simulink model "obstacle_detection"  (R2023a)
settings: Solver=ode1  StartTime=0.0  StopTime=Inf  FixedStep=1/60  RelTol=1e-3
PostLoadFcn:
  | qlabs_setup
model workspace (MAT data in the model file):
  downCamStepSize = Simulink.Parameter
  downCamStepSize.Value = Simulink.data.Expression
  downCamStepSize.Value.ExpressionString = "qc_get_step_size*ceil(1/60/qc_get_step_size)"
  downCamStepSize.DataType = 'auto'
  downCamStepSize.Complexity = 'real'
  downCamStepSize.Dimensions = -1
  lidarStepSize = Simulink.Parameter
  lidarStepSize.Value = Simulink.data.Expression
  lidarStepSize.Value.ExpressionString = "qc_get_step_size*ceil(1/5/qc_get_step_size)"
  lidarStepSize.DataType = 'auto'
  lidarStepSize.Complexity = 'real'
  lidarStepSize.Dimensions = -1
  mainStepSize = Simulink.Parameter
  mainStepSize.Value = Simulink.data.Expression
  mainStepSize.Value.ExpressionString = "qc_get_step_size"
  mainStepSize.DataType = 'auto'
  mainStepSize.Complexity = 'real'
  mainStepSize.Dimensions = -1
  mode = Simulink.Parameter
  mode.Value = 1
  mode.Description = '0 - education speeds via wheel speed commands
    | 1 - education speeds via body speed commands
    | 2 - research speeds via wheel speed commands
    | 3 - research speeds via body speed commands'
  mode.DataType = 'auto'
  mode.Complexity = 'real'
  mode.Dimensions = [1 1]
  realSenseStepSize = Simulink.Parameter
  realSenseStepSize.Value = Simulink.data.Expression
  realSenseStepSize.Value.ExpressionString = "qc_get_step_size*ceil(1/30/qc_get_step_size)"
  realSenseStepSize.DataType = 'auto'
  realSenseStepSize.Complexity = 'real'
  realSenseStepSize.Dimensions = -1
undefined symbols (not defined in the file or in its folder): gcbh, JPEG, Point, video_display_show
libraries: quarc_library x29
settings Model: SimulationMode=external  ExtModeTrigDuration=10000  Creator=mbohra  LastModifiedBy=ZinanCen
settings DebuggingCC: UnderspecifiedInitializationDetection=Classic  MergeDetectMultiDrivingBlocksExec=none
settings ModelReferenceCC: PropagateSignalLabelsOutOfModel=off

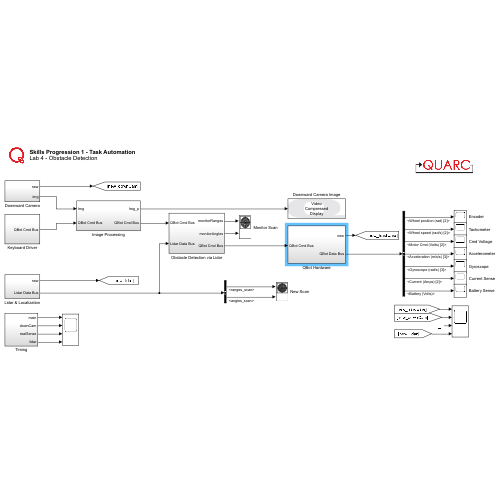
[thumbnail: Simulink's stored preview of the top-level diagram]
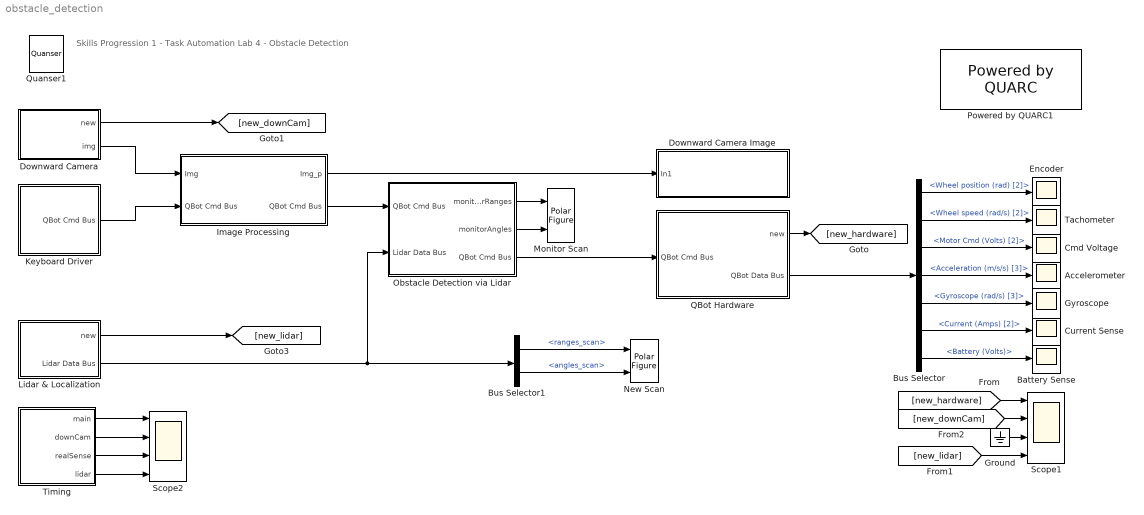
== system obstacle_detection ==
  note: Skills Progression 1 - Task Automation
      | Lab 4 - Obstacle Detection
  Accelerometer : Scope
  Battery Sense : Scope
  Bus Selector : BusSelector  OutputSignals=Wheel position (rad) [2],Wheel speed (rad/s) [2],Motor Cmd (Volts) [2],Acceleration (m/s/s) [3],Gyroscope (rad/s) [3],Current (Amps) [2],Battery (Volts)
  Bus Selector1 : BusSelector  OutputSignals=ranges_scan,angles_scan
  Cmd Voltage : Scope
  Current Sense : Scope
  Downward Camera : Subsystem
  Downward Camera Image : Subsystem  LoadFcn=set_param(gcbh, 'UserData', gcb);  StartFcn=video_display_show([gcb, '/Video Display'], 'add', gcb);  mask(Video Compressed Display){algorithm=JPEG, quality=50, sample_time=-1, use_hardware=on}
      mask prompts: algorithm "Compression algorithm:"; quality "Compression quality (0-100):"; sample_time "Sample time (seconds):"; use_hardware "Use hardware acceleration for video display"
      mask help: Displays a video stream on the host, using compression to minimize bandwidth.
      mask init:
      | qc_set_display('Video\nCompressed\nDisplay');
      settings: UndoDeleteFcn=set_param(gcbh, 'UserData', gcb);  OpenFcn=video_display_show([gcb, '/Video Display'], 'show', gcb);  PreDeleteFcn=video_display_show([gcb, '/Video Display'], 'delete');
      settings: CopyFcn=|
      | set_param(gcbh, 'UserData', gcb);
      | set_param(gcbh, 'LinkStatus', 'none');
      settings: NameChangeFcn=|
      | video_display_show([get_param(gcbh, 'UserData'), '/Video Display'], 'rename', [gcb, '/Video Display']);
      | video_display_show([gcb, '/Video Display'], 'add', gcb);
      | set_param(gcbh, 'UserData', gcb);
      mask Help: web(qc_get_block_help_path(gcb));
      mask TypeOptions algorithm: Image Compress/algorithm
      mask TypeOptions quality: Image Compress/quality
      mask TypeOptions sample_time: Video Display/sample_time
      mask TypeOptions use_hardware: Video Display/use_hardware
      mask Display:
      | patch([0.98591 0.98591 0.62618 0.59072 0.56147   0.536   0.536  0.5441 0.56912 0.59207 0.60881 0.62276 0.63527 0.64364  0.6485  0.6485 0.64706 0.64499 0.63662 0.62411 0.61232 0.59837 0.58307 0.56147   0.536   0.536  0.5441  0.5747 0.60953 0.63662 0.67001  0.7034 0.72851 0.75425 0.77927 0.80294 0.82454 0.84119 0.85865 0.87395 0.88574 0.89339  0.8969 0.89969 0.89969 0.89267  0.8816 0.87044 0.85649  0.8384 0.81824 0.80294 0.78764 0.77513 0.76676 0.75776 0.76397 0.77513 0.79178 0.80987 0.82796 0.84326 0.86207 0.98528],[0.18689 0.05522 0.05522 0.05171 0.05171    0.05 0.18338 0.18338 0.19148 0.20435 0.22298 0.24863 0.28589 0.33125 0.38138 0.55139 0.59801 0.63761 0.68189 0.72149 0.74939 0.76694 0.77855 0.79367 0.79952 0.92768 0.92768 0.92768 0.92417 0.92066 0.91364  0.9032 0.89384 0.88106 0.86594 0.85073 0.82634 0.80537 0.77855 0.74363 0.70403 0.65858 0.61079 0.59099 0.41513 0.37202 0.31847 0.29048 0.25556 0.23342  0.2102 0.19382 0.18221 0.17285 0.16943 0.16124  0.1589 0.16241 0.16709 0.17168  0.1787 0.18221 0.18689 0.18689],[0.9,0.90,0.91])
      | patch([0.536 0.52601 0.46823 0.44528 0.41603 0.39101 0.35555 0.33116 0.31451 0.29291  0.2804 0.26717 0.25322 0.23999 0.22406 0.20732 0.19337 0.17528 0.15935 0.14396 0.13217 0.11759 0.10922 0.10085 0.09671 0.09392 0.09041 0.08906 0.08906 0.09464  0.0995 0.10778 0.11894 0.13145 0.14675 0.16349 0.17672 0.19409 0.20732 0.22406 0.23999 0.26159 0.27833 0.29849 0.31793 0.33602 0.35411 0.37085 0.39245 0.41603   0.536   0.536 0.53159 0.46409   0.446 0.42026 0.39587 0.37571 0.36113 0.34925 0.34088 0.33809 0.33809 0.34088 0.34583 0.35627 0.36392 0.38129 0.39587 0.41117 0.42719 0.44672  0.4676 0.48353 0.48353 0.52394   0.536],[0.05 0.04829 0.04712 0.04712 0.04829 0.05063 0.05405 0.05873 0.06107 0.06692 0.07043 0.07619 0.08087 0.08672 0.09482 0.10652 0.11696 0.13325  0.1508 0.17168 0.19499 0.22415 0.25439 0.28472 0.31379 0.35456 0.38489 0.41513 0.58055 0.63878 0.68774 0.72149 0.75641 0.78089 0.80537 0.82859 0.84029 0.85658 0.86594 0.87404  0.8834 0.89267 0.90086 0.90788 0.91247 0.91832 0.92066   0.923 0.92651 0.92768 0.92768 0.79952 0.79952 0.79952 0.79718 0.78899 0.77153 0.75056 0.72149 0.68072 0.62249  0.5549 0.41396 0.37085 0.33242 0.28121 0.25205 0.22181 0.20552 0.19499 0.18572 0.18221 0.17753 0.17636 0.17753  0.1787  0.1787],[0.9,0.90,0.91])
      | disp('Video\nCompressed\nDisplay');
  Encoder : Scope
  Ground : Ground
  Gyroscope : Scope
  Image Processing : Subsystem
  Keyboard Driver : Subsystem
  Lidar & Localization : Subsystem
  Monitor Scan : quarc_library/Sinks/Figures/Polar Figure  figure_mode=Use figure window  figure_tag=figure1  axes_tag=axes1  plot_mode=Frame-based  minimum_rho=0  maximum_rho=4  minimum_theta=0  maximum_theta=360  zero_location=top  direction=counterclockwise  buffer_size=1  update_rate=1  sample_time=-1  initial_position="1255    81   528   430"  initial_visibility=off  line1_style=None  line1_width=0.5  line1_color=[0 0.4470 0.7410]  marker1=Point (.)  marker1_size=6  marker1_edge_color=[0 0.447059 0.741176]  marker1_face_color=[0 0.447059 0.741176]  line2_style=Solid line (-)  line2_width=0.5  line2_color=[0.85098 0.32549 0.0980392]  marker2=None  marker2_size=6  marker2_edge_color=[0.85098 0.32549 0.0980392]  marker2_face_color=[0.85098 0.32549 0.0980392]  line3_style=Solid line (-)  line3_width=0.5  line3_color=[0.929412 0.694118 0.12549]  marker3=None  marker3_size=6  marker3_edge_color=[0.929412 0.694118 0.12549]  marker3_face_color=[0.929412 0.694118 0.12549]  line4_style=Solid line (-)  line4_width=0.5  line4_color=[0.494118 0.184314 0.556863]  marker4=None  marker4_size=6  marker4_edge_color=[0.494118 0.184314 0.556863]  marker4_face_color=[0.494118 0.184314 0.556863]  line5_style=Solid line (-)  line5_width=0.5  line5_color=[0.466667 0.67451 0.188235]  marker5=None  marker5_size=6  marker5_edge_color=[0.466667 0.67451 0.188235]  marker5_face_color=[0.466667 0.67451 0.188235]
      settings: SourceProductName=QUARC Targets
  New Scan : quarc_library/Sinks/Figures/Polar Figure  figure_mode=Use figure window  figure_tag=figure1  axes_tag=axes1  plot_mode=Frame-based  minimum_rho=0  maximum_rho=4  minimum_theta=0  maximum_theta=360  zero_location=top  direction=counterclockwise  buffer_size=1  update_rate=1  sample_time=-1  initial_position="1256   577   528   426"  initial_visibility=off  line1_style=None  line1_width=0.5  line1_color=[0 0.4470 0.7410]  marker1=Point (.)  marker1_size=6  marker1_edge_color=[0 0.447059 0.741176]  marker1_face_color=[0 0.447059 0.741176]  line2_style=Solid line (-)  line2_width=0.5  line2_color=[0.85098 0.32549 0.0980392]  marker2=None  marker2_size=6  marker2_edge_color=[0.85098 0.32549 0.0980392]  marker2_face_color=[0.85098 0.32549 0.0980392]  line3_style=Solid line (-)  line3_width=0.5  line3_color=[0.929412 0.694118 0.12549]  marker3=None  marker3_size=6  marker3_edge_color=[0.929412 0.694118 0.12549]  marker3_face_color=[0.929412 0.694118 0.12549]  line4_style=Solid line (-)  line4_width=0.5  line4_color=[0.494118 0.184314 0.556863]  marker4=None  marker4_size=6  marker4_edge_color=[0.494118 0.184314 0.556863]  marker4_face_color=[0.494118 0.184314 0.556863]  line5_style=Solid line (-)  line5_width=0.5  line5_color=[0.466667 0.67451 0.188235]  marker5=None  marker5_size=6  marker5_edge_color=[0.466667 0.67451 0.188235]  marker5_face_color=[0.466667 0.67451 0.188235]
      settings: SourceProductName=QUARC Targets
  Obstacle Detection via Lidar : Subsystem
  Powered by QUARC1 : quarc_library/Logos/Powered by QUARC
  QBot Hardware : Subsystem
  Quanser1 : quarc_library/Logos/Quanser
  Scope1 : Scope  NumInputPorts=4
  Scope2 : Scope  NumInputPorts=4
  Tachometer : Scope
  Timing : Subsystem
  wires:
  QBot Hardware/2(QBot Data Bus) -> Bus Selector/1
  QBot Hardware/1(new) -> [new_hardware]
  Bus Selector/1 -> Encoder/1  "<Wheel position (rad) [2]>"
  Bus Selector/3 -> Cmd Voltage/1  "<Motor Cmd (Volts) [2]>"
  Bus Selector/4 -> Accelerometer/1  "<Acceleration (m/s/s) [3]>"
  Bus Selector/6 -> Current Sense/1  "<Current (Amps) [2]>"
  Bus Selector/2 -> Tachometer/1  "<Wheel speed (rad/s) [2]>"
  Bus Selector/5 -> Gyroscope/1  "<Gyroscope (rad/s) [3]>"
  Bus Selector/7 -> Battery Sense/1  "<Battery (Volts)>"
  Lidar & Localization/2(Lidar Data Bus) -> Bus Selector1/1, Obstacle Detection via Lidar/2(Lidar Data Bus)
  Bus Selector1/1 -> New Scan/1  "<ranges_scan>"
  Bus Selector1/2 -> New Scan/2  "<angles_scan>"
  Lidar & Localization/1(new) -> [new_lidar]
  [new_downCam] -> Scope1/2
  Timing/3(realSense) -> Scope2/3
  Timing/4(lidar) -> Scope2/4
  [new_lidar] -> Scope1/4
  Timing/2(downCam) -> Scope2/2
  [new_hardware] -> Scope1/1
  Timing/1(main) -> Scope2/1
  Obstacle Detection via Lidar/1(monitorRanges) -> Monitor Scan/1
  Obstacle Detection via Lidar/2(monitorAngles) -> Monitor Scan/2
  Obstacle Detection via Lidar/3(QBot Cmd Bus) -> QBot Hardware/1(QBot Cmd Bus)
  Downward Camera/2(img) -> Image Processing/1(Img)
  Keyboard Driver/1(QBot Cmd Bus) -> Image Processing/2(QBot Cmd Bus)
  Image Processing/1(Img_p) -> Downward Camera Image/1(In1)
  Image Processing/2(" QBot Cmd Bus") -> Obstacle Detection via Lidar/1("QBot Cmd Bus ")
  Downward Camera/1(new) -> [new_downCam]
  Ground/1 -> Scope1/3

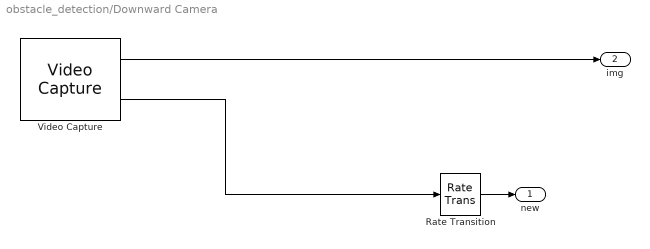
== system obstacle_detection/Downward Camera ==
  Rate Transition : RateTransition
  Video Capture : quarc_library/Multimedia/Video Capture  source=device  device=0@tcpip://localhost:18915  filename=sample_movie.mov  value=[0 0; 0 0]  resolution=640 x 400  width=640  height=400  output_format=MATLAB greyscale (HxW)  data_type=uint8  sample_time=downCamStepSize  brightness_override=off  brightness=50.0  contrast_override=off  contrast=50.0  hue_override=off  hue=50.0  saturation_override=off  saturation=50.0  sharpness_override=off  sharpness=50.0  gamma_override=off  gamma=50.0  coloreffect_override=off  coloreffect=None  whitebalance_override=off  whitebalance=50.0  backlightcompensation_override=off  backlightcompensation=0.0  gain_override=on  gain=17.0  pan_override=off  pan=50.0  tilt_override=off  tilt=50.0  roll_override=off  roll=50.0  zoom_override=off  zoom=0.0  exposure_override=on  exposure=39.0  iris_override=off  iris=50.0  mirror_override=off  mirror=None  focus_override=off  focus=0.0
      settings: SourceProductName=QUARC Targets
  new : Outport
  img : Outport  Port=2
  wires:
  Video Capture/2 -> Rate Transition/1
  Video Capture/1 -> img/1
  Rate Transition/1 -> new/1

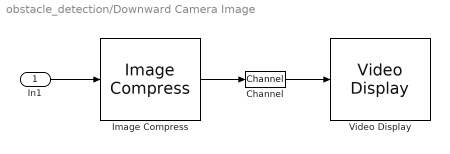
== system obstacle_detection/Downward Camera Image ==
  In1 : Inport
  Channel : quarc_library/Signal Routing/Channel  channel=0  buffer_size=1
  Image Compress : quarc_library/Image Processing/Generic/Image Compress  algorithm=JPEG  source=Internal dialog parameter  quality=quality  output_dim=-1
  Video Display : quarc_library/Multimedia/Video Display  Tag=obstacle_detection_student/Downward Camera Image/Video Display  sample_time=sample_time  use_hardware=on
  wires:
  Channel/1 -> Video Display/1
  In1/1 -> Image Compress/1
  Image Compress/1 -> Channel/1

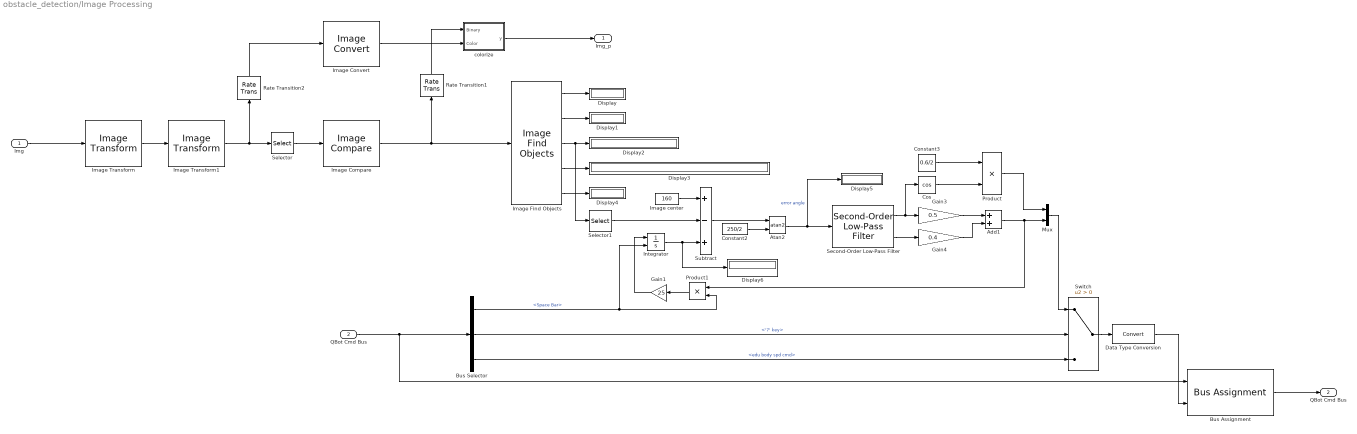
== system obstacle_detection/Image Processing ==
  Img : Inport
  QBot Cmd Bus : Inport  Port=2
  Add1 : Sum
  Atan2 : Trigonometry  Operator=atan2
  Bus Assignment : BusAssignment  AssignedSignals=edu body spd cmd
  Bus Selector : BusSelector  OutputSignals=Space Bar,'7' key,edu body spd cmd
  Constant2 : Constant  Value=250/2
  Constant3 : Constant  Value=0.6/2
  Cos : Trigonometry  Operator=cos
  Data Type Conversion : DataTypeConversion  SaturateOnIntegerOverflow=off  RndMeth=Floor
  Display{,1..6} (7 alike) : Display
      Display settings: Format=bank
      Display1 settings: Format=bank
      Display2 settings: Format=bank
      Display3 settings: Format=bank
      Display4 settings: Format=bank
  Gain1 : Gain  Gain=25
  Gain3 : Gain  Gain=0.5
  Gain4 : Gain  Gain=0.4
  Image Compare : quarc_library/Image Processing/Generic/Image Compare  output_type=Combined (one HxW output)  source=Internal dialog parameters  r_comparison=min <= pixel and pixel <= max  r_minimum=225  r_maximum=255  g_comparison=min <= pixel and pixel <= max  g_minimum=225  g_maximum=255  b_comparison=min <= pixel and pixel <= max  b_minimum=225  b_maximum=255
      settings: SourceProductName=QUARC Targets
  Image Convert : quarc_library/Image Processing/Generic/Image Convert  input_format=MATLAB greyscale (HxW)  padding=0  output_format=MATLAB RGB (HxWx3)  data_type=uint8
      settings: AttributesFormatString=(%<input_format>)  SourceProductName=QUARC Targets
  Image Find Objects : quarc_library/Image Processing/Generic/Image Find Objects  num_objects=1  connectivity=8 directions (N, NE, E, SE, S, SW, W, NW)  sort_order=Sort by number of pixels  min_pixels=500  max_pixels=intmax('uint32')  largest=on  exclude_at_edges=off  variable_size=off  use_complex=off
      settings: SourceProductName=QUARC Targets
  Image Transform : quarc_library/Image Processing/Generic/Image Transform  algorithm=Lens undistort  color_theme=KRYGCBMW  min_pixel=0  max_pixel=4000  focal_length=[302.1629, 301.7493]  principal_point=[185.6271, 306.7551]  radial_coeffs=[-0.3138 0.0780]  tangential_coeffs=[]  extrapolated_pixel=0  interpolation=nearest  row_coords=0  column_coords=0  output_height=480  output_width=640  angle=0  origin=[240 320]  output_origin=[240 320]  output_data_type=uint8
      settings: AttributesFormatString=(%<algorithm>)  SourceProductName=QUARC Targets
  Image Transform1 : quarc_library/Image Processing/Generic/Image Transform  algorithm=Resize  color_theme=KRYGCBMW  min_pixel=0  max_pixel=4000  focal_length=308  principal_point=[262 334]  radial_coeffs=[-0.3129 0.0907]  tangential_coeffs=[]  extrapolated_pixel=0  interpolation=nearest  row_coords=0  column_coords=0  output_height=200  output_width=320  angle=0  origin=[240 320]  output_origin=[240 320]  output_data_type=uint8
      settings: AttributesFormatString=(%<algorithm>)  SourceProductName=QUARC Targets
  Image center : Constant  Value=160
  Integrator : Integrator  ExternalReset=falling  LimitOutput=on  UpperSaturationLimit=75  LowerSaturationLimit=-75
  Mux : Mux  Inputs=2
  Product : Product
  Product1 : Product
  Rate Transition1 : RateTransition  OutPortSampleTime=downCamStepSize*2
  Rate Transition2 : RateTransition  OutPortSampleTime=downCamStepSize*2
  Second-Order Low-Pass Filter : quarc_library/Continuous/Second-Order Low-Pass Filter  params_source=Internal (dialog parameters)  input_width=2*pi*5  input_zeta=1  input_init=0
  Selector : Selector  NumberOfDimensions=2  InputPortWidth=3  IndexOptions=Index vector (dialog),Select all  Indices=[51:100],[101:540]  OutputSizes=1,1
  Selector1 : Selector  InputPortWidth=2  IndexOptions=Index vector (dialog)  Indices=2  OutputSizes=1
  Subtract : Sum  Inputs=+-+
  Switch : Switch  Criteria=u2 > Threshold  SaturateOnIntegerOverflow=off  InputSameDT=off
  colorize : MATLAB Function  TreatAsAtomicUnit=on
  Img_p : Outport
  " QBot Cmd Bus" : Outport  Port=2
  wires:
  Selector1/1 -> Subtract/2
  Image center/1 -> Subtract/1
  Image Find Objects/5 -> Display4/1
  Image Find Objects/3 -> Display2/1, Selector1/1
  Image Find Objects/4 -> Display3/1
  Image Find Objects/2 -> Display1/1
  Image Find Objects/1 -> Display/1
  Image Compare/1 -> Image Find Objects/1, Rate Transition1/1
  Image Transform1/1 -> Rate Transition2/1, Selector/1
  Selector/1 -> Image Compare/1
  Rate Transition1/1 -> colorize/1(Binary)
  Atan2/1 -> Display5/1, Second-Order Low-Pass Filter/1  "error angle"
  Subtract/1 -> Atan2/1
  Constant2/1 -> Atan2/2
  Cos/1 -> Product/2
  Constant3/1 -> Product/1
  Product/1 -> Mux/1
  Mux/1 -> Switch/1
  Add1/1 -> Product1/1, Mux/2
  Integrator/1 -> Display6/1, Subtract/3
  Gain1/1 -> Integrator/1
  Bus Selector/1 -> Integrator/2, Product1/2  "<Space Bar>"
  Gain4/1 -> Add1/2
  Gain3/1 -> Add1/1
  Second-Order Low-Pass Filter/2 -> Gain4/1
  Second-Order Low-Pass Filter/1 -> Cos/1, Gain3/1
  Product1/1 -> Gain1/1
  Rate Transition2/1 -> Image Convert/1
  colorize/1(y) -> Img_p/1
  Image Convert/1 -> colorize/2(Color)
  Image Transform/1 -> Image Transform1/1
  Img/1 -> Image Transform/1
  QBot Cmd Bus/1 -> Bus Assignment/1, Bus Selector/1
  Bus Selector/3 -> Switch/3  "<edu body spd cmd>"
  Bus Selector/2 -> Switch/2  "<'7' key>"
  Switch/1 -> Data Type Conversion/1
  Bus Assignment/1 -> " QBot Cmd Bus"/1
  Data Type Conversion/1 -> Bus Assignment/2

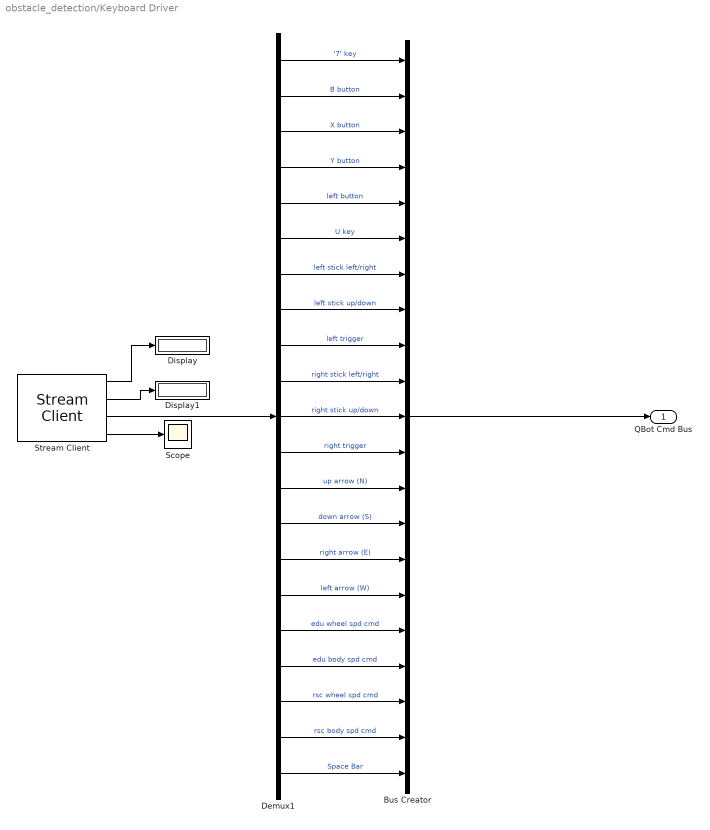
== system obstacle_detection/Keyboard Driver ==
  Bus Creator : BusCreator  Inputs=21
  Demux1 : Demux  Outputs=[1 1 1 1 1 1 1 1 1 1 1 1 1 1 1 1 2 2 2 2 1]
  Display : Display
  Display1 : Display
  Scope : Scope
  Stream Client : quarc_library/Communications/Basic/Stream Client  uri_source=Specify via dialog (do not evaluate)  uri=tcpip://localhost:18889?nagle='off'  send_buffer_size=1460  receive_buffer_size=1460  byte_order=little endian (Intel - LSB first)  optimization=Minimum latency  send_options=Do not send data  receive_options=Receive most recent data  default_value=zeros(25,1)  sample_time=qc_get_step_size  active=on  implementation=Use blocking I/O in a separate thread  send_fifo_size=1000  receive_fifo_size=1000  send_priority=0  receive_priority=0  send_dimensions=off  receive_dimensions=off  max_dimensions=-1  data_type=Inherited via back propagation  type_expr=BusObject
      settings: AttributesFormatString="\"tcpip://localhost:18889?nagle='off'\""
  QBot Cmd Bus : Outport
  wires:
  Bus Creator/1 -> QBot Cmd Bus/1
  Stream Client/3 -> Demux1/1
  Demux1/1 -> Bus Creator/1  "'7' key"
  Demux1/2 -> Bus Creator/2  "B button"
  Demux1/3 -> Bus Creator/3  "X button"
  Demux1/4 -> Bus Creator/4  "Y button"
  Demux1/5 -> Bus Creator/5  "left button"
  Demux1/6 -> Bus Creator/6  "U key"
  Demux1/7 -> Bus Creator/7  "left stick left/right"
  Demux1/8 -> Bus Creator/8  "left stick up/down"
  Demux1/9 -> Bus Creator/9  "left trigger"
  Demux1/10 -> Bus Creator/10  "right stick left/right"
  Demux1/11 -> Bus Creator/11  "right stick up/down"
  Demux1/12 -> Bus Creator/12  "right trigger"
  Demux1/13 -> Bus Creator/13  "up arrow (N)"
  Demux1/14 -> Bus Creator/14  "down arrow (S)"
  Demux1/15 -> Bus Creator/15  "right arrow (E)"
  Demux1/16 -> Bus Creator/16  "left arrow (W)"
  Demux1/17 -> Bus Creator/17  "edu wheel spd cmd"
  Demux1/18 -> Bus Creator/18  "edu body spd cmd"
  Demux1/19 -> Bus Creator/19  "rsc wheel spd cmd"
  Demux1/20 -> Bus Creator/20  "rsc body spd cmd"
  Demux1/21 -> Bus Creator/21  "Space Bar"
  Stream Client/1 -> Display/1
  Stream Client/2 -> Display1/1
  Stream Client/4 -> Scope/1

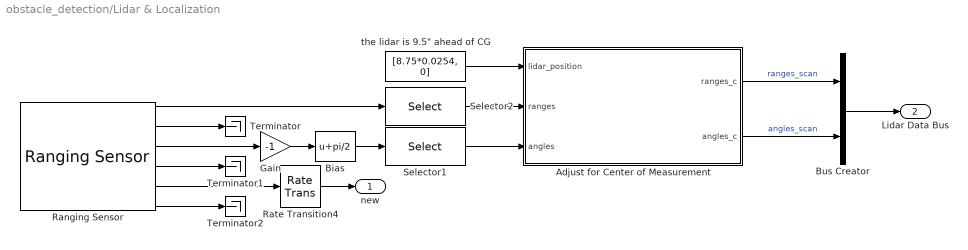
== system obstacle_detection/Lidar & Localization ==
  Adjust for Center of Measurement : MATLAB Function  TreatAsAtomicUnit=on
  Bias : Bias  Bias=pi/2  SaturateOnIntegerOverflow=off
  Bus Creator : BusCreator  Inputs=2
  Gain : Gain  Gain=-1
  Ranging Sensor : quarc_library/Devices/Third-Party/Sensors/Ranging Sensor  sensor_type=Leishen M10P LIDAR  uri=tcpip://localhost:18918  ranging_distance=Short  timing_budget=0.033  measurement_period=0.0005  output_mode=Fixed-size output  samples_per_revolution=1680  max_distance=0.050  max_angle=5  sample_time=lidarStepSize  show_versions=off  active=on
      settings: SourceProductName=QUARC Targets
  Rate Transition4 : RateTransition
  Selector1 : Selector  InputPortWidth=1680  IndexOptions=Index vector (dialog)  Indices=[1:4:1677]  OutputSizes=1
  Selector2 : Selector  InputPortWidth=1680  IndexOptions=Index vector (dialog)  Indices=[1:4:1677]  OutputSizes=1
  Terminator : Terminator
  Terminator1 : Terminator
  Terminator2 : Terminator
  "the lidar is 9.5\" ahead of CG" : Constant  Value=[8.75*0.0254, 0]  SampleTime=lidarStepSize
  new : Outport
  Lidar Data Bus : Outport  Port=2
  wires:
  Ranging Sensor/5 -> Rate Transition4/1
  Rate Transition4/1 -> new/1
  Selector1/1 -> Adjust for Center of Measurement/3(angles)
  Selector2/1 -> Adjust for Center of Measurement/2(ranges)
  "the lidar is 9.5\" ahead of CG"/1 -> Adjust for Center of Measurement/1(lidar_position)
  Bias/1 -> Selector1/1
  Ranging Sensor/2 -> Terminator/1
  Ranging Sensor/4 -> Terminator1/1
  Gain/1 -> Bias/1
  Ranging Sensor/3 -> Gain/1
  Ranging Sensor/1 -> Selector2/1
  Bus Creator/1 -> Lidar Data Bus/1
  Ranging Sensor/6 -> Terminator2/1
  Adjust for Center of Measurement/1(ranges_c) -> Bus Creator/1  "ranges_scan"
  Adjust for Center of Measurement/2(angles_c) -> Bus Creator/2  "angles_scan"

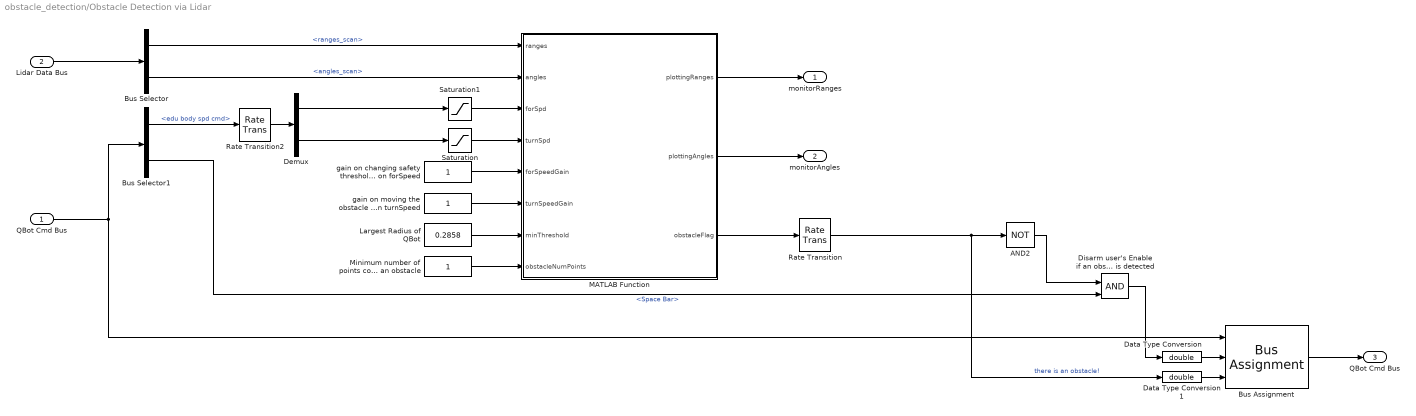
== system obstacle_detection/Obstacle Detection via Lidar ==
  "QBot Cmd Bus " : Inport
  Lidar Data Bus : Inport  Port=2
  AND2 : Logic  Operator=NOT  IconShape=distinctive  AllPortsSameDT=off  OutDataTypeStr=boolean
  Bus Assignment : BusAssignment  AssignedSignals=Space Bar,Y button
  Bus Selector : BusSelector  OutputSignals=ranges_scan,angles_scan
  Bus Selector1 : BusSelector  OutputSignals=edu body spd cmd,Space Bar
  Data Type Conversion : DataTypeConversion  OutDataTypeStr=double  SaturateOnIntegerOverflow=off  RndMeth=Floor
  Data Type Conversion1 : DataTypeConversion  OutDataTypeStr=double  SaturateOnIntegerOverflow=off  RndMeth=Floor
  Demux : Demux  Outputs=2
  Disarm user's Enable if an obstacle is detected : Logic  IconShape=distinctive  AllPortsSameDT=off  OutDataTypeStr=boolean
  Largest Radius of QBot : Constant  Value=0.2858
  MATLAB Function : MATLAB Function  TreatAsAtomicUnit=on
  Minimum number of points considered as an obstacle : Constant
  Rate Transition : RateTransition
  Rate Transition2 : RateTransition
  Saturation : Saturate  UpperLimit=3.564  LowerLimit=-3.564
  Saturation1 : Saturate  UpperLimit=0.35  LowerLimit=-0.35
  gain on changing safety threshold based on forSpeed : Constant
  "gain on moving the obstacle scan area left and right based on turnSpeed " : Constant
  monitorRanges : Outport
  monitorAngles : Outport  Port=2
  QBot Cmd Bus : Outport  Port=3
  wires:
  Lidar Data Bus/1 -> Bus Selector/1
  Bus Selector/1 -> MATLAB Function/1(ranges)  "<ranges_scan>"
  Bus Selector/2 -> MATLAB Function/2(angles)  "<angles_scan>"
  Bus Selector1/1 -> Rate Transition2/1  "<edu body spd cmd>"
  Saturation1/1 -> MATLAB Function/3(forSpd)
  MATLAB Function/3(obstacleFlag) -> Rate Transition/1
  Demux/2 -> Saturation/1
  Minimum number of points considered as an obstacle/1 -> MATLAB Function/8(obstacleNumPoints)
  Demux/1 -> Saturation1/1
  MATLAB Function/1(plottingRanges) -> monitorRanges/1
  MATLAB Function/2(plottingAngles) -> monitorAngles/1
  "QBot Cmd Bus "/1 -> Bus Selector1/1, Bus Assignment/1
  Saturation/1 -> MATLAB Function/4(turnSpd)
  Rate Transition2/1 -> Demux/1
  AND2/1 -> Disarm user's Enable if an obstacle is detected/1
  Bus Selector1/2 -> Disarm user's Enable if an obstacle is detected/2  "<Space Bar>"
  Bus Assignment/1 -> QBot Cmd Bus/1
  Disarm user's Enable if an obstacle is detected/1 -> Data Type Conversion/1
  Rate Transition/1 -> Data Type Conversion1/1, AND2/1  "there is an obstacle!"
  Data Type Conversion/1 -> Bus Assignment/2
  Data Type Conversion1/1 -> Bus Assignment/3
  "gain on moving the obstacle scan area left and right based on turnSpeed "/1 -> MATLAB Function/6(turnSpeedGain)
  Largest Radius of QBot/1 -> MATLAB Function/7(minThreshold)
  gain on changing safety threshold based on forSpeed/1 -> MATLAB Function/5(forSpeedGain)

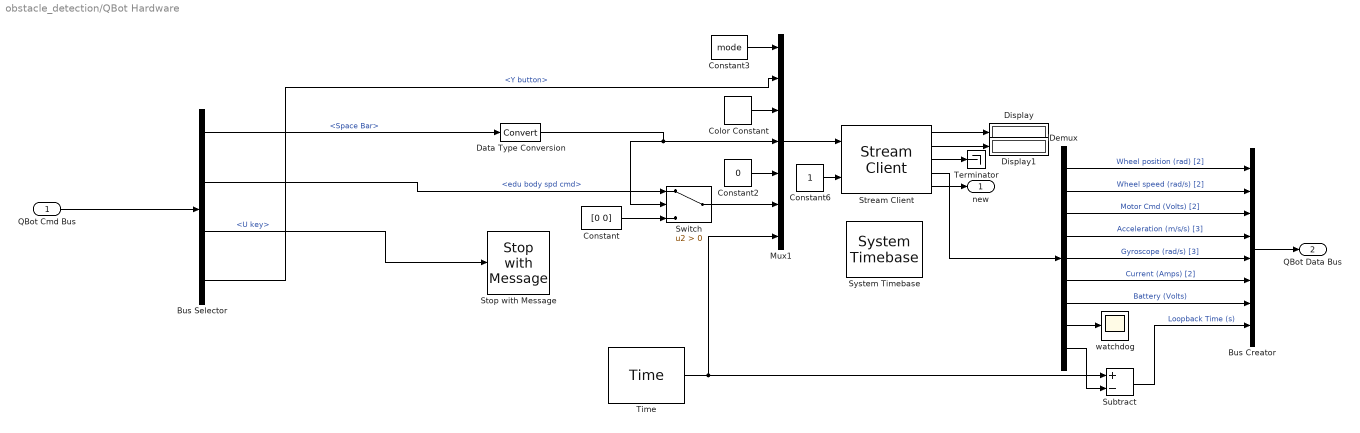
== system obstacle_detection/QBot Hardware ==
  QBot Cmd Bus : Inport
  Bus Creator : BusCreator  Inputs=8
  Bus Selector : BusSelector  OutputSignals=Space Bar,edu body spd cmd,U key,Y button
  Color Constant : quarc_library/Sources/Signals/Color Constant  color=[1 0 1]
      settings: SourceProductName=QUARC Targets
  Constant : Constant  Value=[0 0]
  Constant2 : Constant  Value=0
  Constant3 : Constant  Value=mode
  Constant6 : Constant
  Data Type Conversion : DataTypeConversion  SaturateOnIntegerOverflow=off  RndMeth=Floor
  Demux : Demux  Outputs=[2 2 2 3 3 2 1 1 1]
  Display : Display
  Display1 : Display
  Mux1 : Mux  Inputs=7
  Stop with Message : quarc_library/Sinks/Error Handling/Stop with Message  message_type=Fixed error message  message_icon=Information  message=Operator: Emergency Stop
  Stream Client : quarc_library/Communications/Basic/Stream Client  uri_source=Specify via dialog (do not evaluate)  uri=tcpip://localhost:18888  send_buffer_size=1460  receive_buffer_size=1460  byte_order=little endian (Intel - LSB first)  optimization=Minimum latency  send_options=Send most recent data  receive_options=Receive most recent data  default_value=zeros(17,1)  sample_time=qc_get_step_size  active=on  implementation=Use blocking I/O in a separate thread  send_fifo_size=1000  receive_fifo_size=1000  send_priority=0  receive_priority=0  send_dimensions=off  receive_dimensions=off  max_dimensions=-1  data_type=Inherited via back propagation  type_expr=BusObject
      settings: AttributesFormatString="\"tcpip://localhost:18888\""
  Subtract : Sum  Inputs=+-
  Switch : Switch  Criteria=u2 > Threshold  SaturateOnIntegerOverflow=off  InputSameDT=off
  System Timebase : quarc_library/Advanced/Timing/System Timebase  stop_on_overrun=off
      settings: SourceProductName=QUARC Targets
  Terminator : Terminator
  Time : quarc_library/Sources/Time/Time  time_source=Wall clock  sample_time=qc_get_step_size
  watchdog : Scope
  new : Outport
  QBot Data Bus : Outport  Port=2
  wires:
  Demux/2 -> Bus Creator/2  "Wheel speed (rad/s) [2]"
  Constant3/1 -> Mux1/1
  Stream Client/3 -> Terminator/1
  Bus Selector/2 -> Switch/1  "<edu body spd cmd>"
  Stream Client/1 -> Display/1
  Constant6/1 -> Stream Client/2
  Stream Client/2 -> Display1/1
  Color Constant/1 -> Mux1/3
  Demux/3 -> Bus Creator/3  "Motor Cmd (Volts) [2]"
  Mux1/1 -> Stream Client/1
  Stream Client/4 -> Demux/1
  Demux/1 -> Bus Creator/1  "Wheel position (rad) [2]"
  Stream Client/5 -> new/1
  Demux/7 -> Bus Creator/7  "Battery (Volts)"
  Demux/5 -> Bus Creator/5  "Gyroscope (rad/s) [3]"
  Demux/6 -> Bus Creator/6  "Current (Amps) [2]"
  Demux/9 -> Subtract/2
  Constant2/1 -> Mux1/5
  Demux/4 -> Bus Creator/4  "Acceleration (m/s/s) [3]"
  Time/1 -> Mux1/7, Subtract/1
  Bus Creator/1 -> QBot Data Bus/1
  Subtract/1 -> Bus Creator/8  "Loopback Time (s)"
  Demux/8 -> watchdog/1
  Switch/1 -> Mux1/6
  Constant/1 -> Switch/3
  QBot Cmd Bus/1 -> Bus Selector/1
  Bus Selector/3 -> Stop with Message/1  "<U key>"
  Bus Selector/1 -> Data Type Conversion/1  "<Space Bar>"
  Data Type Conversion/1 -> Switch/2, Mux1/4
  Bus Selector/4 -> Mux1/2  "<Y button>"

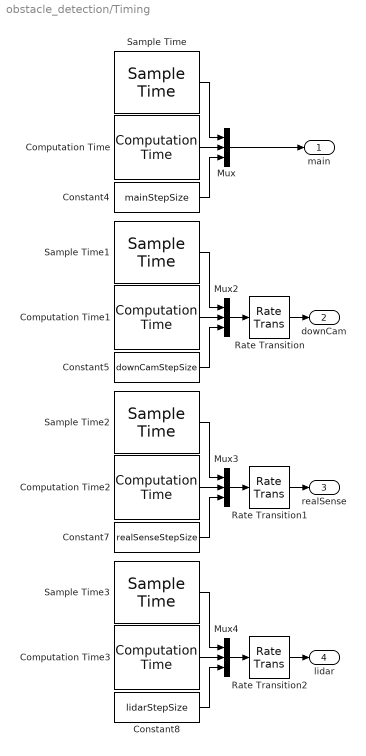
== system obstacle_detection/Timing ==
  Computation Time : quarc_library/Sources/Time/Computation Time  sample_time=mainStepSize  use_model=on  use_cpu_time=off
  Computation Time1 : quarc_library/Sources/Time/Computation Time  sample_time=downCamStepSize  use_model=on  use_cpu_time=off
  Computation Time2 : quarc_library/Sources/Time/Computation Time  sample_time=realSenseStepSize  use_model=on  use_cpu_time=off
  Computation Time3 : quarc_library/Sources/Time/Computation Time  sample_time=lidarStepSize  use_model=on  use_cpu_time=off
  Constant4 : Constant  Value=mainStepSize
  Constant5 : Constant  Value=downCamStepSize
  Constant7 : Constant  Value=realSenseStepSize
  Constant8 : Constant  Value=lidarStepSize
  Mux{,2..4} (4 alike) : Mux  Inputs=3
  Rate Transition : RateTransition
  Rate Transition1 : RateTransition
  Rate Transition2 : RateTransition
  Sample Time : quarc_library/Sources/Time/Sample Time  Priority=-99  sample_time=mainStepSize
  Sample Time1 : quarc_library/Sources/Time/Sample Time  Priority=-99  sample_time=downCamStepSize
  Sample Time2 : quarc_library/Sources/Time/Sample Time  Priority=-99  sample_time=realSenseStepSize
  Sample Time3 : quarc_library/Sources/Time/Sample Time  Priority=-99  sample_time=lidarStepSize
  main : Outport
  downCam : Outport  Port=2
  realSense : Outport  Port=3
  lidar : Outport  Port=4
  wires:
  Rate Transition1/1 -> realSense/1
  Computation Time2/1 -> Mux3/2
  Constant5/1 -> Mux2/3
  Mux4/1 -> Rate Transition2/1
  Computation Time/1 -> Mux/2
  Sample Time/1 -> Mux/1
  Constant8/1 -> Mux4/3
  Sample Time1/1 -> Mux2/1
  Mux3/1 -> Rate Transition1/1
  Computation Time1/1 -> Mux2/2
  Constant4/1 -> Mux/3
  Mux2/1 -> Rate Transition/1
  Computation Time3/1 -> Mux4/2
  Sample Time2/1 -> Mux3/1
  Constant7/1 -> Mux3/3
  Sample Time3/1 -> Mux4/1
  Rate Transition/1 -> downCam/1
  Rate Transition2/1 -> lidar/1
  Mux/1 -> main/1

== matlab function obstacle_detection/Obstacle Detection via Lidar/MATLAB Function ==
  data: ranges input; plottingRanges output; angles input; forSpd input; turnSpd input; forSpeedGain input; plottingAngles output; turnSpeedGain input; minThreshold input; obstacleNumPoints input; obstacleFlag output
function [plottingRanges, plottingAngles, obstacleFlag] = detect_obstacle(ranges, angles, forSpd, turnSpd, forSpeedGain, turnSpeedGain, minThreshold, obstacleNumPoints)
    
    
    
    
    halfNumPoints = 205;
    quarterNumPoints = round(halfNumPoints/2);
    % Grab the first half of ranges and angles representing 180 degrees
    frontRanges = ranges(1:halfNumPoints);
    frontAngles = angles(1:halfNumPoints);
    % Starting index in top half          1     West
    % Mid point in west quadrant         51     North-west
    % Center index in top half          102     North
    % Mid point in east quadrant     51+102     North-east
    % Ending index in top half          205     East

    
    % Section 1 - Dynamic Focus Region
    
    %-------Replace the following line with your code---------%

    % Determine the start of the focus region 
    startingIndex = 1;

    %---------------------------------------------------------%

    
    monitorRanges = frontRanges(startingIndex:startingIndex+quarterNumPoints);
    monitorAngles = frontAngles(startingIndex:startingIndex+quarterNumPoints);

    
    % Section 2 - Dynamic Stop Distance

    %-------Replace the following line with your code---------%

    % Determine safetyThreshold based on Forward Speed 
    safetyThreshold = 1;

    %---------------------------------------------------------%
    
    % At angles corresponding to monitorAngles, pick uniform ranges based on
    % a safety threshold
    safetyAngles = monitorAngles;
    safetyRanges = safetyThreshold*monitorRanges./monitorRanges;

   
    % Section 3 - Obstacle Detection

    %-------Replace the following line with your code---------%

    % Total number of obstacles detected between 
    % minThreshold & safetyThreshold
    % Then determin obstacleFlag based on totalObstaclePoints
    totalObstaclePoints = 0;
    obstacleFlag = 0;

    %---------------------------------------------------------%

    
    % Lidar Ranges and Angles for plotting (both scan & safety zone)
    plottingRanges = [monitorRanges; safetyRanges];
    plottingAngles = [monitorAngles; safetyAngles];

end

== matlab function obstacle_detection/Lidar & Localization/Adjust for Center of Measurement ==
  data: lidar_position input; ranges input; ranges_c output; angles input; angles_c output
function [ranges_c,angles_c] = correct_lidar(lidar_position, ranges,angles)

% Convert lidar data from polar into cartesian, and add lidar position
% Then Convert back into polar coordinates
%-------Replace the following line with your code---------%
ranges_c = ranges;
angles_c = angles./angles;
%---------------------------------------------------------%
end

== matlab function obstacle_detection/Image Processing/colorize ==
  data: Binary input; y output; Color input
function y = fcn(Binary, Color)

y = Color;
[ROW, COL, ~] = size(y);

y(51:100, 1:COL, 1) = ((255 - Binary)/255).*Color(51:100,:,1) + (Binary).*Color(51:100, :, 1);
y(51:100, 1:COL, 2) = ((255 - Binary)/255).*Color(51:100,:,2);
y(51:100, 1:COL, 3) = ((255 - Binary)/255).*Color(51:100,:,3);
